simulink model "Simulink_Audio"  (R2021b)
settings: Solver=VariableStepAuto  StartTime=0.0  StopTime=Inf  RelTol=1e-3
libraries: dspsigops x2, dspsrcs4 x2, dspsnks4 x1, dspvision x1
settings Model: Creator=enrique  LastModifiedBy=enrique
settings SolverCC: AlgebraicLoopSolver=TrustRegion
settings DebuggingCC: SFMachineParentedDataDiag=warning

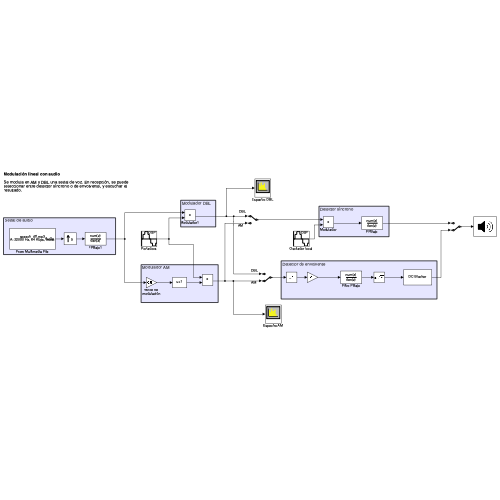
[thumbnail: Simulink's stored preview of the top-level diagram]
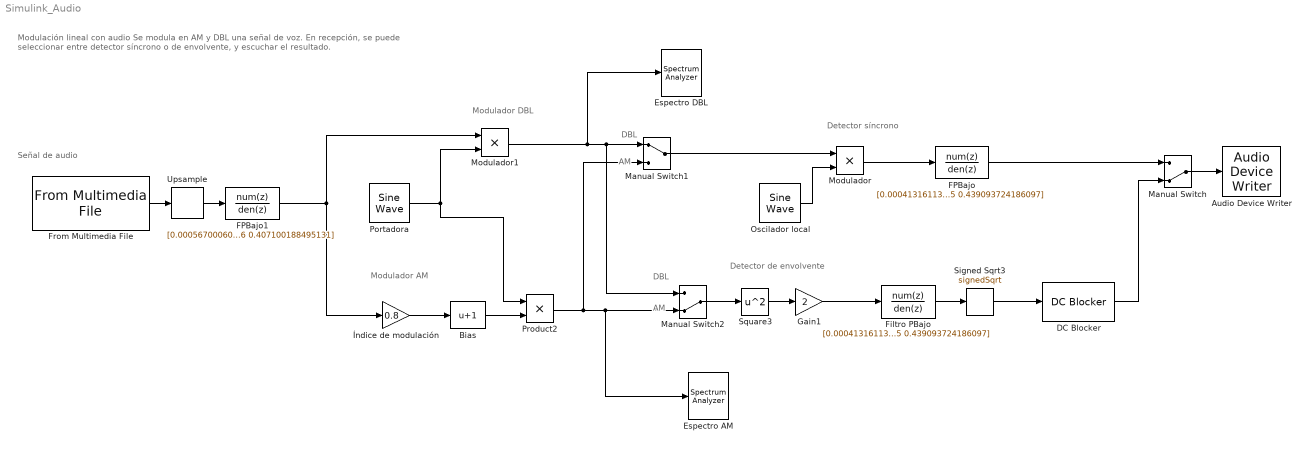
== system Simulink_Audio ==
  note: Modulación lineal con audio
      |
      | Se modula en AM y DBL una señal de voz. En recepción, se puede seleccionar entre detector síncrono o de envolvente, y escuchar el resultado.
  note: DBL
  note: Modulador DBL
  note: Detector síncrono
  note: Señal de audio
  note: Detector de envolvente
  note: Modulador AM
  note: DBL
  note: AM
  note: AM
  Audio Device Writer : dspsnks4/Audio Device Writer  Driver=CoreAudio  Device=Default  InheritSampleRate=on  SampleRate=44100  BitDepth=16-bit integer  BufferSize=4096  NumBuffers=10  DefaultOutputChannelMapping=on  OutputChannelMapping=1:2  OutputNumUnderrunSamples=off  DriverIdx=5  DeviceWarnFlag=''
  Bias : Bias  Bias=1
  DC Blocker : dspsigops/DC Blocker  Algorithm=IIR  NormalizedBandwidth=0.001  Length=8  Order=6  SimulateUsing=Code generation
      settings: SourceProductBaseCode=DS
  Espectro AM : SpectrumAnalyzer
  Espectro DBL : SpectrumAnalyzer
  FPBajo : DiscreteFilter  Numerator="[0.000413161134215036\t0.00165264453686014\t0.00247896680529022\t0.00165264453686014\t0.000413161134215036]"  Denominator="[1\t-3.18248964930004\t3.86534233322133\t-2.11533582995995\t0.439093724186097]"  InputProcessing=Columns as channels (frame based)
  FPBajo1 : DiscreteFilter  Numerator="[0.000567000605622080\t0.00226800242248832\t0.00340200363373248\t0.00226800242248832\t0.000567000605622080]"  Denominator="[1\t-3.10848114066775\t3.70178606768923\t-1.99133310582666\t0.407100188495131]"  InputProcessing=Columns as channels (frame based)
  Filtro PBajo : DiscreteFilter  Numerator="[0.000413161134215036\t0.00165264453686014\t0.00247896680529022\t0.00165264453686014\t0.000413161134215036]"  Denominator="[1\t-3.18248964930004\t3.86534233322133\t-2.11533582995995\t0.439093724186097]"  InputProcessing=Columns as channels (frame based)
  From Multimedia File : dspvision/From Multimedia File  inputFilename=/Applications/MATLAB_R2021b.app/toolbox/dsp/dsp/speech_dft.mp3  readRange=[1 Inf]  loop=on  numPlays=Inf  outputStreams=Audio only  videoDataType=single  audioDataType=double  inheritSampleTime=on  userDefinedSampleTime=1/30  noAudioOutput=off  isIntensityVideo=off  fourcc=RGB  colorVideoFormat=Separate color signals  outputEOF=off  dataOrg=Column-major  audioFrameSize=1024  computeAudioFrameSize=off  outSamplingMode=Sample based
  Gain1 : Gain  Gain=2
  Manual Switch : ManualSwitch  CurrentSetting=0
  Manual Switch1 : ManualSwitch
  Manual Switch2 : ManualSwitch  CurrentSetting=0
  Modulador : Product  OutDataTypeStr=Inherit: Same as first input
  Modulador1 : Product  OutDataTypeStr=Inherit: Same as first input
  Oscilador local : dspsrcs4/Sine Wave  Amplitude=1  Frequency=30000  Phase=0  SampleMode=Discrete  OutComplex=Real  CompMethod=Trigonometric fcn  TableSize=Speed  SampleTime=1/(22050*5)  SamplesPerFrame=1024*5  ResetState=Catch up to simulation time  OutputFrames=off  dataType=double  wordLen=16  udDataType=sfix(16)  fracBitsMode=Best precision  numFracBits=15  OutDataTypeStr=double  LastOutDataTypeStr=double
  Portadora : dspsrcs4/Sine Wave  Amplitude=1  Frequency=30000  Phase=0  SampleMode=Discrete  OutComplex=Real  CompMethod=Trigonometric fcn  TableSize=Speed  SampleTime=1/(22050*5)  SamplesPerFrame=1024*5  ResetState=Catch up to simulation time  OutputFrames=off  dataType=double  wordLen=16  udDataType=sfix(16)  fracBitsMode=Best precision  numFracBits=15  OutDataTypeStr=double  LastOutDataTypeStr=double
  Product2 : Product  OutDataTypeStr=Inherit: Same as first input
  Signed Sqrt3 : Sqrt  Operator=signedSqrt  SaturateOnIntegerOverflow=on
  Square3 : Math  Operator=square  SaturateOnIntegerOverflow=on
  Upsample : dspsigops/Upsample  N=5  phase=0  InputProcessing=Columns as channels (frame based)  RateOptions=Enforce single-rate processing  ic=0  mode=Unused parameter value
  "Índice de modulación " : Gain  Gain=0.8
  wires:
  From Multimedia File/1 -> Upsample/1
  Upsample/1 -> FPBajo1/1
  Oscilador local/1 -> Modulador/2
  Modulador/1 -> FPBajo/1
  Portadora/1 -> Modulador1/2, Product2/1
  Filtro PBajo/1 -> Signed Sqrt3/1
  Gain1/1 -> Filtro PBajo/1
  Square3/1 -> Gain1/1
  "Índice de modulación "/1 -> Bias/1
  FPBajo1/1 -> Modulador1/1, "Índice de modulación "/1
  Bias/1 -> Product2/2
  Signed Sqrt3/1 -> DC Blocker/1
  Manual Switch/1 -> Audio Device Writer/1
  FPBajo/1 -> Manual Switch/1
  DC Blocker/1 -> Manual Switch/2
  Modulador1/1 -> Espectro DBL/1, Manual Switch2/1, Manual Switch1/1
  Product2/1 -> Espectro AM/1, Manual Switch2/2, Manual Switch1/2
  Manual Switch1/1 -> Modulador/1
  Manual Switch2/1 -> Square3/1
